simulink model "sistemviza1"  (R2016a)
settings: Solver=VariableStepAuto  StartTime=0.0  StopTime=350  RelTol=1e-3
values from neighbouring files (symbols this model uses):
  Ag = 0.8    [Valori.m]
  Dg = 0    [Valori.m]
  Gb = 80    [Valori.m]
  n = 0.109    [Valori.m]
  p1 = 0.029    [Valori.m]
  p2 = 0.029    [Valori.m]
  p3 = 0.00000783    (= 7.83e-06)    [Valori.m]
  tgmax = 40    [Valori.m]
  V = 120    [Valori.m]
  Xb = 0.0054    [Valori.m]
settings Model: Creator=carme  LastModifiedBy=carme

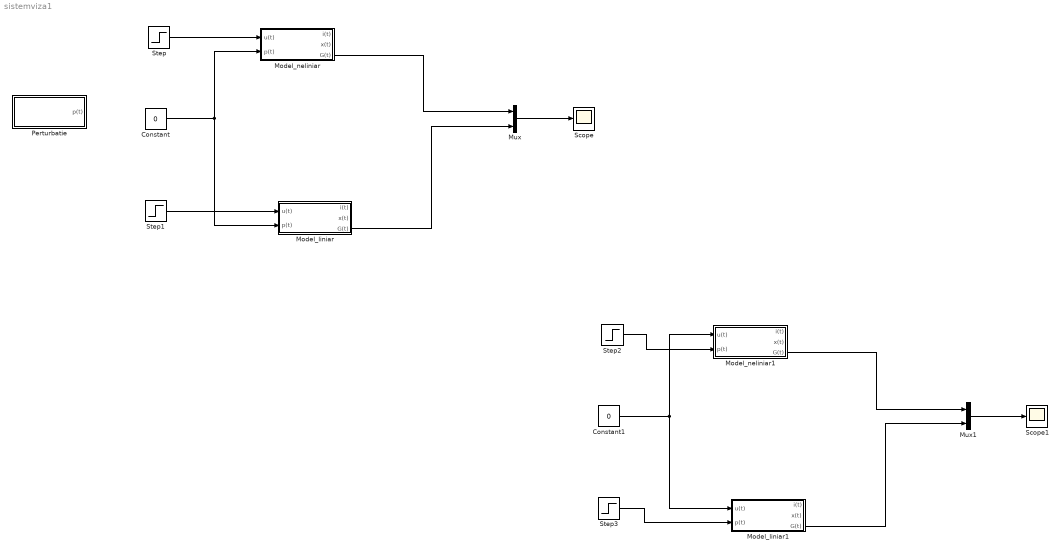
== system sistemviza1 ==
  Constant : Constant  Value=0
  Constant1 : Constant  Value=0
  Model_liniar : Subsystem
  Model_liniar1 : Subsystem
  Model_neliniar : Subsystem
  Model_neliniar1 : Subsystem
  Mux : Mux  Inputs=2
  Mux1 : Mux  Inputs=2
  Perturbatie : Subsystem
  Scope : Scope
  Scope1 : Scope
  Step{,1..3} (4 alike) : Step  SampleTime=0
  wires:
  Mux/1 -> Scope/1
  Step/1 -> Model_neliniar/1(u(t))
  Constant/1 -> Model_neliniar/2(p(t)), Model_liniar/2(p(t))
  Step1/1 -> Model_liniar/1(u(t))
  Model_liniar/3(G(t)) -> Mux/2
  Model_neliniar/3(G(t)) -> Mux/1
  Mux1/1 -> Scope1/1
  Model_liniar1/3(G(t)) -> Mux1/2
  Model_neliniar1/3(G(t)) -> Mux1/1
  Constant1/1 -> Model_neliniar1/1(u(t)), Model_liniar1/1(u(t))
  Step3/1 -> Model_liniar1/2(p(t))
  Step2/1 -> Model_neliniar1/2(p(t))

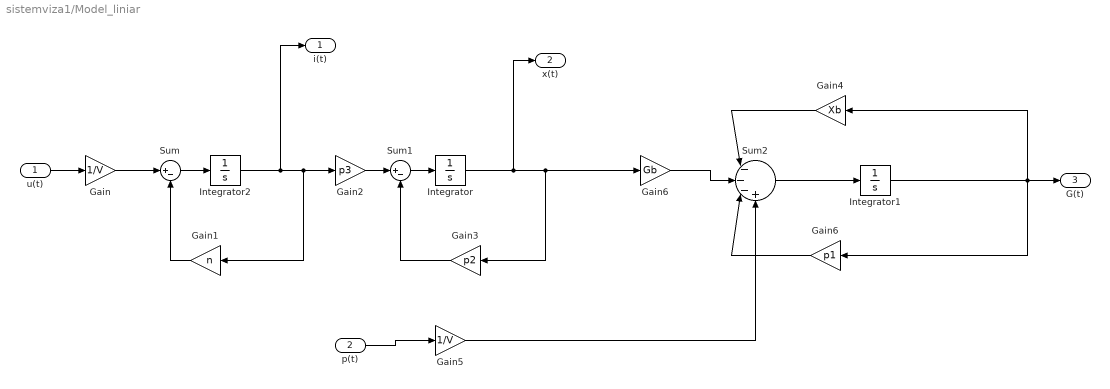
== system sistemviza1/Model_liniar ==
  u(t) : Inport
  p(t) : Inport  Port=2
  Gain : Gain  Gain=1/V
  Gain1 : Gain  Gain=n
  Gain2 : Gain  Gain=p3
  Gain3 : Gain  Gain=p2
  Gain4 : Gain  Gain=Xb
  Gain5 : Gain  Gain=1/V
  Gain6 : Gain  Gain=p1
  "Gain6 " : Gain  Gain=Gb
  Integrator : Integrator
  Integrator1 : Integrator  InitialCondition=300
  Integrator2 : Integrator
  Sum : Sum  Inputs=|+-
  Sum1 : Sum  Inputs=|+-
  Sum2 : Sum  Inputs=|---+
  i(t) : Outport
  x(t) : Outport  Port=2
  G(t) : Outport  Port=3
  wires:
  u(t)/1 -> Gain/1
  Gain/1 -> Sum/1
  Sum/1 -> Integrator2/1
  Integrator2/1 -> i(t)/1, Gain1/1, Gain2/1
  Gain2/1 -> Sum1/1
  Sum1/1 -> Integrator/1
  Gain1/1 -> Sum/2
  Gain3/1 -> Sum1/2
  Integrator/1 -> x(t)/1, Gain3/1, "Gain6 "/1
  p(t)/1 -> Gain5/1
  Gain5/1 -> Sum2/4
  "Gain6 "/1 -> Sum2/2
  Sum2/1 -> Integrator1/1
  Integrator1/1 -> Gain4/1, Gain6/1, G(t)/1
  Gain4/1 -> Sum2/1
  Gain6/1 -> Sum2/3

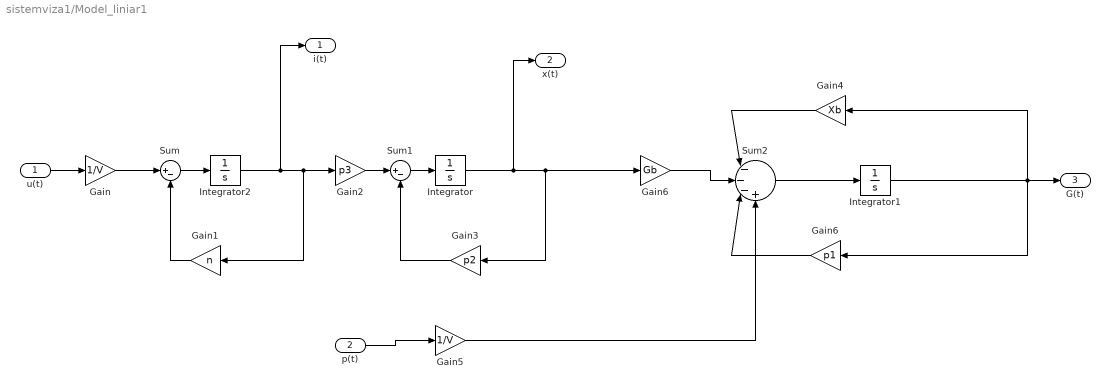
== system sistemviza1/Model_liniar1 ==
  u(t) : Inport
  p(t) : Inport  Port=2
  Gain : Gain  Gain=1/V
  Gain1 : Gain  Gain=n
  Gain2 : Gain  Gain=p3
  Gain3 : Gain  Gain=p2
  Gain4 : Gain  Gain=Xb
  Gain5 : Gain  Gain=1/V
  Gain6 : Gain  Gain=p1
  "Gain6 " : Gain  Gain=Gb
  Integrator : Integrator
  Integrator1 : Integrator  InitialCondition=80
  Integrator2 : Integrator
  Sum : Sum  Inputs=|+-
  Sum1 : Sum  Inputs=|+-
  Sum2 : Sum  Inputs=|---+
  i(t) : Outport
  x(t) : Outport  Port=2
  G(t) : Outport  Port=3
  wires:
  u(t)/1 -> Gain/1
  Gain/1 -> Sum/1
  Sum/1 -> Integrator2/1
  Integrator2/1 -> i(t)/1, Gain1/1, Gain2/1
  Gain2/1 -> Sum1/1
  Sum1/1 -> Integrator/1
  Gain1/1 -> Sum/2
  Gain3/1 -> Sum1/2
  Integrator/1 -> x(t)/1, Gain3/1, "Gain6 "/1
  p(t)/1 -> Gain5/1
  Gain5/1 -> Sum2/4
  "Gain6 "/1 -> Sum2/2
  Sum2/1 -> Integrator1/1
  Integrator1/1 -> Gain4/1, Gain6/1, G(t)/1
  Gain4/1 -> Sum2/1
  Gain6/1 -> Sum2/3

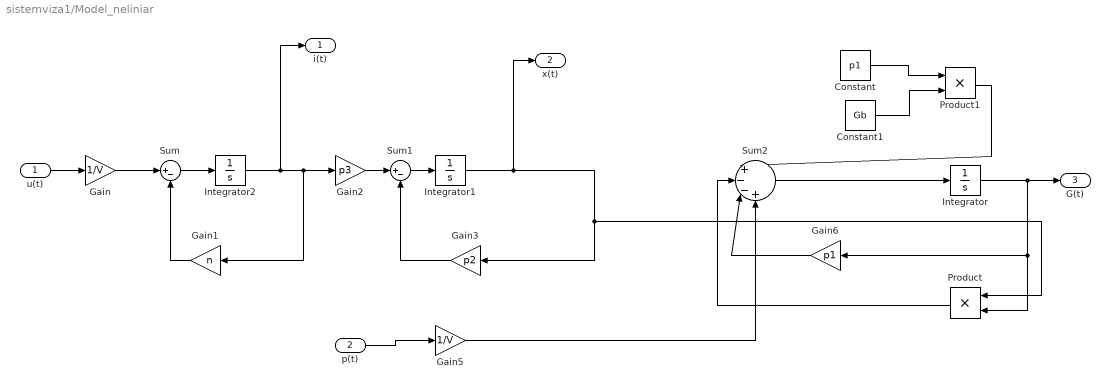
== system sistemviza1/Model_neliniar ==
  u(t) : Inport
  p(t) : Inport  Port=2
  Constant : Constant  Value=p1
  Constant1 : Constant  Value=Gb
  Gain : Gain  Gain=1/V
  Gain1 : Gain  Gain=n
  Gain2 : Gain  Gain=p3
  Gain3 : Gain  Gain=p2
  Gain5 : Gain  Gain=1/V
  Gain6 : Gain  Gain=p1
  Integrator : Integrator  InitialCondition=300
  Integrator1 : Integrator
  Integrator2 : Integrator
  Product : Product
  Product1 : Product
  Sum : Sum  Inputs=|+-
  Sum1 : Sum  Inputs=|+-
  Sum2 : Sum  Inputs=|+--+
  i(t) : Outport
  x(t) : Outport  Port=2
  G(t) : Outport  Port=3
  wires:
  u(t)/1 -> Gain/1
  Gain/1 -> Sum/1
  Sum/1 -> Integrator2/1
  Integrator2/1 -> i(t)/1, Gain1/1, Gain2/1
  Gain2/1 -> Sum1/1
  Sum1/1 -> Integrator1/1
  Gain1/1 -> Sum/2
  Gain3/1 -> Sum1/2
  Integrator1/1 -> x(t)/1, Product/1, Gain3/1
  p(t)/1 -> Gain5/1
  Gain5/1 -> Sum2/4
  Integrator/1 -> Product/2, Gain6/1, G(t)/1
  Gain6/1 -> Sum2/3
  Constant/1 -> Product1/1
  Constant1/1 -> Product1/2
  Product1/1 -> Sum2/1
  Product/1 -> Sum2/2
  Sum2/1 -> Integrator/1

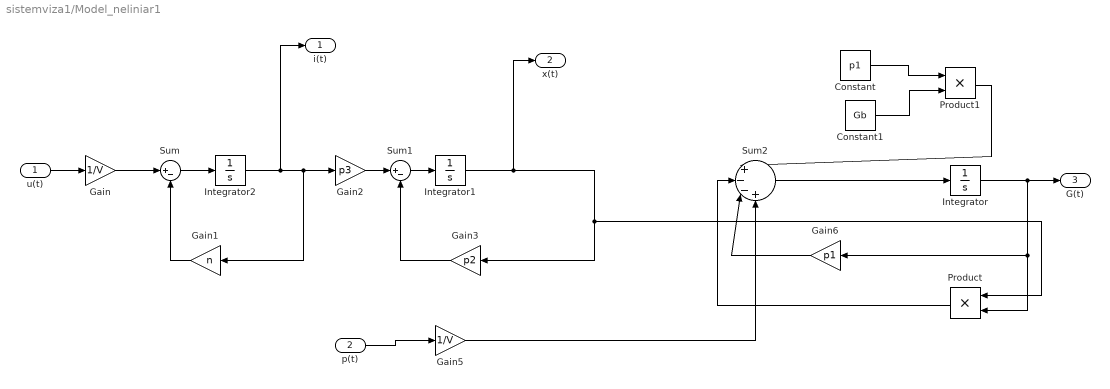
== system sistemviza1/Model_neliniar1 ==
  u(t) : Inport
  p(t) : Inport  Port=2
  Constant : Constant  Value=p1
  Constant1 : Constant  Value=Gb
  Gain : Gain  Gain=1/V
  Gain1 : Gain  Gain=n
  Gain2 : Gain  Gain=p3
  Gain3 : Gain  Gain=p2
  Gain5 : Gain  Gain=1/V
  Gain6 : Gain  Gain=p1
  Integrator : Integrator  InitialCondition=80
  Integrator1 : Integrator
  Integrator2 : Integrator
  Product : Product
  Product1 : Product
  Sum : Sum  Inputs=|+-
  Sum1 : Sum  Inputs=|+-
  Sum2 : Sum  Inputs=|+--+
  i(t) : Outport
  x(t) : Outport  Port=2
  G(t) : Outport  Port=3
  wires:
  u(t)/1 -> Gain/1
  Gain/1 -> Sum/1
  Sum/1 -> Integrator2/1
  Integrator2/1 -> i(t)/1, Gain1/1, Gain2/1
  Gain2/1 -> Sum1/1
  Sum1/1 -> Integrator1/1
  Gain1/1 -> Sum/2
  Gain3/1 -> Sum1/2
  Integrator1/1 -> x(t)/1, Product/1, Gain3/1
  p(t)/1 -> Gain5/1
  Gain5/1 -> Sum2/4
  Integrator/1 -> Product/2, Gain6/1, G(t)/1
  Gain6/1 -> Sum2/3
  Constant/1 -> Product1/1
  Constant1/1 -> Product1/2
  Product1/1 -> Sum2/1
  Product/1 -> Sum2/2
  Sum2/1 -> Integrator/1

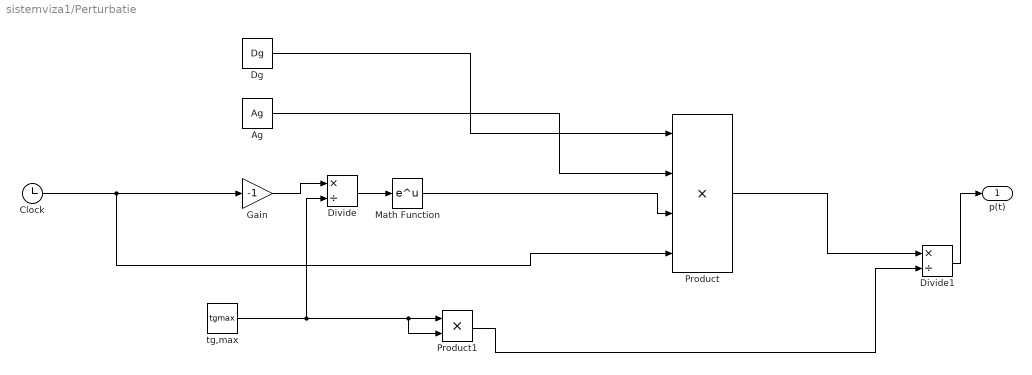
== system sistemviza1/Perturbatie ==
  Ag : Constant  Value=Ag
  "Clock " : Clock
  Dg : Constant  Value=Dg
  Divide : Product  Inputs=*/
  Divide1 : Product  Inputs=*/
  Gain : Gain  Gain=-1
  Math Function : Math  SaturateOnIntegerOverflow=on
  Product : Product  Inputs=4
  Product1 : Product
  tg,max : Constant  Value=tgmax
  p(t) : Outport
  wires:
  Dg/1 -> Product/1
  Ag/1 -> Product/2
  Math Function/1 -> Product/3
  "Clock "/1 -> Product/4, Gain/1
  tg,max/1 -> Divide/2, Product1/2, Product1/1
  Divide/1 -> Math Function/1
  Gain/1 -> Divide/1
  Product1/1 -> Divide1/2
  Divide1/1 -> p(t)/1
  Product/1 -> Divide1/1
